simulink library "halout"  (R2021b)
settings: Solver=VariableStepAuto  StartTime=0.0  StopTime=10.0  RelTol=1e-3
undefined symbols (not defined in the file): C_TASK_5MS_S, FALSE, KHAL_CAN1FD1APS3E2E_flg, KHAL_CAN1FD1APS3TxReq_flg, KHAL_CAN1FD1VCU2E2E_flg, KHAL_CAN1FD1VCU2TxReq_flg, KHAL_CAN1FD1VCU3E2E_flg, KHAL_CAN1FD1VCU3TxReq_flg, KHAL_CAN1TxReq_flg, KHAL_CAN1VMCFCM1E2E_flg, KHAL_CAN1VMCFCM1TxReq_flg, KHAL_CAN2TxReq_flg, KHAL_CAN3FD3VCU1toNIDECTxReq_flg, KHAL_CAN3FD3VCU1TxReq_flg, KHAL_CAN3FD3VCU2E2E_flg, KHAL_CAN3FD3VCU2toNIDECE2E_flg, KHAL_CAN3FD3VCU2toNIDECTxReq_flg, KHAL_CAN3FD3VCU2TxReq_flg, KHAL_CAN3TxReq_flg, KHAL_CAN4FD4CE1000E2E_flg, KHAL_CAN4FD4CE1000TxReq_flg, KHAL_CAN4TxReq_flg, KHAL_CAN5TxReq_flg, KHAL_CAN6FD6APS3E2E_flg, KHAL_CAN6FD6APS3TxReq_flg, KHAL_CAN6FD6VCU2E2E_flg, KHAL_CAN6FD6VCU2TxReq_flg, KHAL_CAN6TxReq_flg, ONE_INT, TRUE, ZERO_INT
libraries: FVT_lib x500, simulink x235
(part 6 of 25)

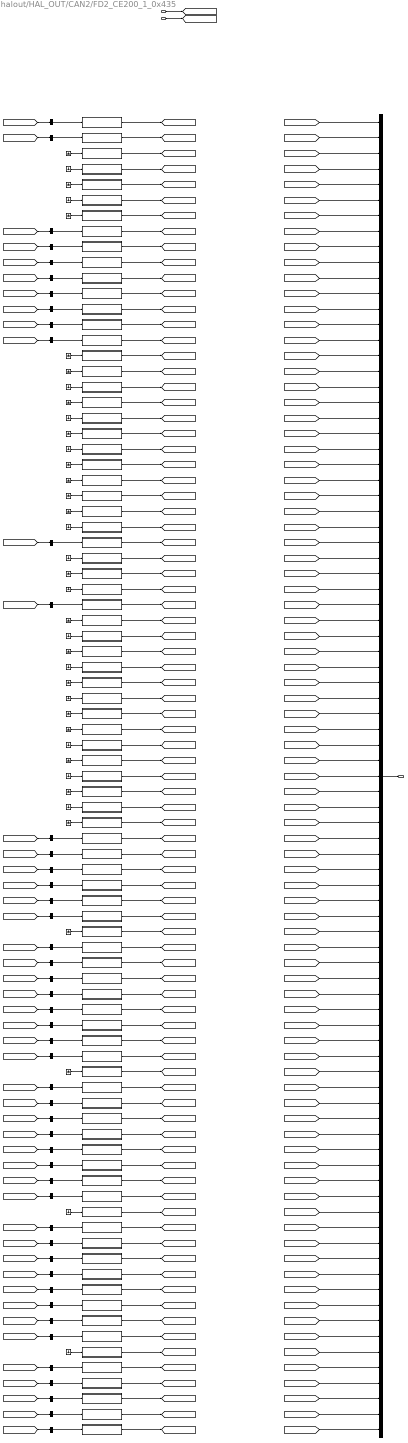
== system halout/HAL_OUT/CAN2/FD2_CE200_1_0x435 ==
  BSCP_outputs : Inport  OutDataTypeStr=Bus: BSCP_outputs
  BOUTP_outputs : Inport  Port=2  OutDataTypeStr=Bus: BOUTP_outputs
  AutoLTips : Subsystem
  CWheelTips : Subsystem
  FDCBCMAcc1StaSta : Subsystem
  FDCBCMAcc2StaSta : Subsystem
  FDCBCMAcc3StaSta : Subsystem
  FDCBCMAcc4StaSta : Subsystem
  FDCBCMAcc5StaSta : Subsystem
  FDCBCMAmbBrightStaSta : Subsystem
  FDCBCMAmbColorStaSta : Subsystem
  FDCBCMAmbDimENSta : Subsystem
  FDCBCMAmbFunENSta : Subsystem
  FDCBCMAmbLinkDriStaSta : Subsystem
  FDCBCMAmbODAENSta : Subsystem
  FDCBCMAmbPwrWarnENSta : Subsystem
  FDCBCMAmbWelENSta : Subsystem
  FDCBCMCLWinLockDrSta : Subsystem
  FDCBCMFollowMeENFunSta : Subsystem
  FDCBCMKey10AccSta : Subsystem
  FDCBCMKey1AccSta : Subsystem
  FDCBCMKey2AccSta : Subsystem
  FDCBCMKey3AccSta : Subsystem
  FDCBCMKey4AccSta : Subsystem
  FDCBCMKey5AccSta : Subsystem
  FDCBCMKey6AccSta : Subsystem
  FDCBCMKey7AccSta : Subsystem
  FDCBCMKey8AccSta : Subsystem
  FDCBCMKey9AccSta : Subsystem
  FDCBCMLockAlarmCmd : Subsystem
  FDCBCMPTGOpenHeightSta : Subsystem
  FDCBCMRmLpModeENFunSta : Subsystem
  FDCBCMTurnSwTSetStaSta : Subsystem
  FDCBCMUserNowSta : Subsystem
  FDCBCMWalkInUnLkEnFunSta : Subsystem
  FDCBCMWalkOutLkEnFunSta : Subsystem
  FDCDKCDkeyShowIVISta : Subsystem
  FDCDKCKeyMissSta : Subsystem
  FDCDKCKeyNumSta : Subsystem
  FDCDKCKeyTypeSta : Subsystem
  FDCDKCUIDLowPowerSta : Subsystem
  FDCFGSAirIntSta : Subsystem
  FDCFGSFGSChSta : Subsystem
  FDCFGSIONSWSta : Subsystem
  FDCSPTGSPTGENFunSta : Subsystem
  FDCTHCMAPTCForceOFFSta : Subsystem
  FDCTHCMAPTCWarningSta : Subsystem
  FDCTHCMAirIntZ3Sta : Subsystem
  Ground{,1..37} (38 alike) : Ground
  LFBatWarn : Subsystem
  LFPressIndi : Subsystem
  LFSensorFail : Subsystem
  LFWheelDebug : Subsystem
  LFWheelPSW : Subsystem
  LFWheelPress : Subsystem
  LFWheelShield : Subsystem
  LFWheelTemp : Subsystem
  LFWheelTmpIndi : Subsystem
  LRBatWarn : Subsystem
  LRPressIndi : Subsystem
  LRSensorFail : Subsystem
  LRWheelDebug : Subsystem
  LRWheelPSW : Subsystem
  LRWheelPress : Subsystem
  LRWheelShield : Subsystem
  LRWheelTemp : Subsystem
  LRWheelTmpIndi : Subsystem
  RFBatWarn : Subsystem
  RFPressIndi : Subsystem
  RFSensorFail : Subsystem
  RFWheelDebug : Subsystem
  RFWheelPSW : Subsystem
  RFWheelPress : Subsystem
  RFWheelShield : Subsystem
  RFWheelTemp : Subsystem
  RFWheelTmpIndi : Subsystem
  RRBatWarn : Subsystem
  RRPressIndi : Subsystem
  RRSensorFail : Subsystem
  RRWheelDebug : Subsystem
  RRWheelPSW : Subsystem
  RRWheelPress : Subsystem
  RRWheelShield : Subsystem
  RRWheelTemp : Subsystem
  RRWheelTmpIndi : Subsystem
  TPMSCaliButtAllow : Subsystem
  TPMSResButtAllow : Subsystem
  TPMSWarnIndi : Subsystem
  bus_creator : BusCreator  Inputs=85  OutDataTypeStr=Bus: DT_CAN2_SG_FD2_CE200_1  NonVirtualBus=on
  bus_selector : BusSelector  OutputSignals=VOUTP_AutoLTips_enum
  bus_selector1 : BusSelector  OutputSignals=VOUTP_CWheelTips_enum
  bus_selector10 : BusSelector  OutputSignals=VOUTP_LockAlarm_enum
  bus_selector11 : BusSelector  OutputSignals=VOUTP_UserNow_enum
  bus_selector12 : BusSelector  OutputSignals=VOUTP_LFBatWarn_flg
  bus_selector13 : BusSelector  OutputSignals=VOUTP_LFPressIndi_enum
  bus_selector14 : BusSelector  OutputSignals=VOUTP_LFSensorFail_flg
  bus_selector15 : BusSelector  OutputSignals=VOUTP_LFWheelDebug_flg
  bus_selector16 : BusSelector  OutputSignals=VOUTP_LFWheelPSW_raw8
  bus_selector17 : BusSelector  OutputSignals=VOUTP_LFWheelPress_raw8
  bus_selector18 : BusSelector  OutputSignals=VOUTP_LFWheelTemp_C
  bus_selector19 : BusSelector  OutputSignals=VOUTP_LFWheelTmpIndi_flg
  bus_selector2 : BusSelector  OutputSignals=VOUTP_AmbBrightSta_enum
  bus_selector20 : BusSelector  OutputSignals=VOUTP_LRBatWarn_flg
  bus_selector21 : BusSelector  OutputSignals=VOUTP_LRPressIndi_enum
  bus_selector22 : BusSelector  OutputSignals=VOUTP_LRSensorFail_flg
  bus_selector23 : BusSelector  OutputSignals=VOUTP_LRWheelDebug_flg
  bus_selector24 : BusSelector  OutputSignals=VOUTP_LRWheelPSW_raw8
  bus_selector25 : BusSelector  OutputSignals=VOUTP_LRWheelPress_raw8
  bus_selector26 : BusSelector  OutputSignals=VOUTP_LRWheelTemp_C
  bus_selector27 : BusSelector  OutputSignals=VOUTP_LRWheelTmpIndi_flg
  bus_selector28 : BusSelector  OutputSignals=VOUTP_RFBatWarn_flg
  bus_selector29 : BusSelector  OutputSignals=VOUTP_RFPressIndi_enum
  bus_selector3 : BusSelector  OutputSignals=VOUTP_AmbColorSta_enum
  bus_selector30 : BusSelector  OutputSignals=VOUTP_RFSensorFail_flg
  bus_selector31 : BusSelector  OutputSignals=VOUTP_RFWheelDebug_flg
  bus_selector32 : BusSelector  OutputSignals=VOUTP_RFWheelPSW_raw8
  bus_selector33 : BusSelector  OutputSignals=VOUTP_RFWheelPress_raw8
  bus_selector34 : BusSelector  OutputSignals=VOUTP_RFWheelTemp_C
  bus_selector35 : BusSelector  OutputSignals=VOUTP_RFWheelTmpIndi_flg
  bus_selector36 : BusSelector  OutputSignals=VOUTP_RRBatWarn_flg
  bus_selector37 : BusSelector  OutputSignals=VOUTP_RRPressIndi_enum
  bus_selector38 : BusSelector  OutputSignals=VOUTP_RRSensorFail_flg
  bus_selector39 : BusSelector  OutputSignals=VOUTP_RRWheelDebug_flg
  bus_selector4 : BusSelector  OutputSignals=VOUTP_AmbDimEN_flg
  bus_selector40 : BusSelector  OutputSignals=VOUTP_RRWheelPSW_raw8
  bus_selector41 : BusSelector  OutputSignals=VOUTP_RRWheelPress_raw8
  bus_selector42 : BusSelector  OutputSignals=VOUTP_RRWheelTemp_C
  bus_selector43 : BusSelector  OutputSignals=VOUTP_RRWheelTmpIndi_flg
  bus_selector44 : BusSelector  OutputSignals=VOUTP_TPMSWarnIndi_enum
  bus_selector45 : BusSelector  OutputSignals=VOUTP_TPMSCaliButtAllow_flg
  bus_selector46 : BusSelector  OutputSignals=VOUTP_TPMSResButtAllow_flg
  bus_selector5 : BusSelector  OutputSignals=VOUTP_AmbFunEN_flg
  bus_selector6 : BusSelector  OutputSignals=VOUTP_AmbLinkDriSta_flg
  bus_selector7 : BusSelector  OutputSignals=VOUTP_AmbODAEN_flg
  bus_selector8 : BusSelector  OutputSignals=VOUTP_AmbPwrWarnEN_flg
  bus_selector9 : BusSelector  OutputSignals=VOUTP_AmbWelEN_flg
  FD2_CE200_1 : Outport
  wires:
  BSCP_outputs/1 -> [BSCP_outputs]
  BOUTP_outputs/1 -> [BOUTP_outputs]
  [CAN2_AutoLTips] -> bus_creator/1  "CAN2_AutoLTips"
  [CAN2_CWheelTips] -> bus_creator/2  "CAN2_CWheelTips"
  [CAN2_FDC_BCM_Acc1Sta_Sta] -> bus_creator/3  "CAN2_FDC_BCM_Acc1Sta_Sta"
  [CAN2_FDC_BCM_Acc2Sta_Sta] -> bus_creator/4  "CAN2_FDC_BCM_Acc2Sta_Sta"
  [CAN2_FDC_BCM_Acc3Sta_Sta] -> bus_creator/5  "CAN2_FDC_BCM_Acc3Sta_Sta"
  [CAN2_FDC_BCM_Acc4Sta_Sta] -> bus_creator/6  "CAN2_FDC_BCM_Acc4Sta_Sta"
  [CAN2_FDC_BCM_Acc5Sta_Sta] -> bus_creator/7  "CAN2_FDC_BCM_Acc5Sta_Sta"
  [CAN2_FDC_BCM_AmbBrightSta_Sta] -> bus_creator/8  "CAN2_FDC_BCM_AmbBrightSta_Sta"
  [CAN2_FDC_BCM_AmbColorSta_Sta] -> bus_creator/9  "CAN2_FDC_BCM_AmbColorSta_Sta"
  [CAN2_FDC_BCM_AmbDimEN_Sta] -> bus_creator/10  "CAN2_FDC_BCM_AmbDimEN_Sta"
  [CAN2_FDC_BCM_AmbFunEN_Sta] -> bus_creator/11  "CAN2_FDC_BCM_AmbFunEN_Sta"
  [CAN2_FDC_BCM_AmbLinkDriSta_Sta] -> bus_creator/12  "CAN2_FDC_BCM_AmbLinkDriSta_Sta"
  [CAN2_FDC_BCM_AmbODAEN_Sta] -> bus_creator/13  "CAN2_FDC_BCM_AmbODAEN_Sta"
  [CAN2_FDC_BCM_AmbPwrWarnEN_Sta] -> bus_creator/14  "CAN2_FDC_BCM_AmbPwrWarnEN_Sta"
  [CAN2_FDC_BCM_AmbWelEN_Sta] -> bus_creator/15  "CAN2_FDC_BCM_AmbWelEN_Sta"
  [CAN2_FDC_BCM_CLWinLockDr_Sta] -> bus_creator/16  "CAN2_FDC_BCM_CLWinLockDr_Sta"
  [CAN2_FDC_BCM_FollowMeENFun_Sta] -> bus_creator/17  "CAN2_FDC_BCM_FollowMeENFun_Sta"
  [CAN2_FDC_BCM_Key10Acc_Sta] -> bus_creator/18  "CAN2_FDC_BCM_Key10Acc_Sta"
  [CAN2_FDC_BCM_Key1Acc_Sta] -> bus_creator/19  "CAN2_FDC_BCM_Key1Acc_Sta"
  [CAN2_FDC_BCM_Key2Acc_Sta] -> bus_creator/20  "CAN2_FDC_BCM_Key2Acc_Sta"
  [CAN2_FDC_BCM_Key3Acc_Sta] -> bus_creator/21  "CAN2_FDC_BCM_Key3Acc_Sta"
  [CAN2_FDC_BCM_Key4Acc_Sta] -> bus_creator/22  "CAN2_FDC_BCM_Key4Acc_Sta"
  [CAN2_FDC_BCM_Key5Acc_Sta] -> bus_creator/23  "CAN2_FDC_BCM_Key5Acc_Sta"
  [CAN2_FDC_BCM_Key6Acc_Sta] -> bus_creator/24  "CAN2_FDC_BCM_Key6Acc_Sta"
  [CAN2_FDC_BCM_Key7Acc_Sta] -> bus_creator/25  "CAN2_FDC_BCM_Key7Acc_Sta"
  [CAN2_FDC_BCM_Key8Acc_Sta] -> bus_creator/26  "CAN2_FDC_BCM_Key8Acc_Sta"
  [CAN2_FDC_BCM_Key9Acc_Sta] -> bus_creator/27  "CAN2_FDC_BCM_Key9Acc_Sta"
  [CAN2_FDC_BCM_LockAlarm_Cmd] -> bus_creator/28  "CAN2_FDC_BCM_LockAlarm_Cmd"
  [CAN2_FDC_BCM_PTGOpenHeight_Sta] -> bus_creator/29  "CAN2_FDC_BCM_PTGOpenHeight_Sta"
  [CAN2_FDC_BCM_RmLpModeENFun_Sta] -> bus_creator/30  "CAN2_FDC_BCM_RmLpModeENFun_Sta"
  [CAN2_FDC_BCM_TurnSwTSetSta_Sta] -> bus_creator/31  "CAN2_FDC_BCM_TurnSwTSetSta_Sta"
  [CAN2_FDC_BCM_UserNow_Sta] -> bus_creator/32  "CAN2_FDC_BCM_UserNow_Sta"
  [CAN2_FDC_BCM_WalkInUnLkEnFun_Sta] -> bus_creator/33  "CAN2_FDC_BCM_WalkInUnLkEnFun_Sta"
  [CAN2_FDC_BCM_WalkOutLkEnFun_Sta] -> bus_creator/34  "CAN2_FDC_BCM_WalkOutLkEnFun_Sta"
  [CAN2_FDC_DKC_DkeyShowIVI_Sta] -> bus_creator/35  "CAN2_FDC_DKC_DkeyShowIVI_Sta"
  [CAN2_FDC_DKC_KeyMiss_Sta] -> bus_creator/36  "CAN2_FDC_DKC_KeyMiss_Sta"
  [CAN2_FDC_DKC_KeyNum_Sta] -> bus_creator/37  "CAN2_FDC_DKC_KeyNum_Sta"
  [CAN2_FDC_DKC_KeyType_Sta] -> bus_creator/38  "CAN2_FDC_DKC_KeyType_Sta"
  [CAN2_FDC_DKC_UIDLowPower_Sta] -> bus_creator/39  "CAN2_FDC_DKC_UIDLowPower_Sta"
  [CAN2_FDC_FGS_AirInt_Sta] -> bus_creator/40  "CAN2_FDC_FGS_AirInt_Sta"
  [CAN2_FDC_FGS_FGSCh_Sta] -> bus_creator/41  "CAN2_FDC_FGS_FGSCh_Sta"
  [CAN2_FDC_FGS_IONSW_Sta] -> bus_creator/42  "CAN2_FDC_FGS_IONSW_Sta"
  [CAN2_FDC_SPTG_SPTGENFun_Sta] -> bus_creator/43  "CAN2_FDC_SPTG_SPTGENFun_Sta"
  [CAN2_FDC_THCM_APTCForceOFF_Sta] -> bus_creator/44  "CAN2_FDC_THCM_APTCForceOFF_Sta"
  [CAN2_FDC_THCM_APTCWarning_Sta] -> bus_creator/45  "CAN2_FDC_THCM_APTCWarning_Sta"
  [CAN2_FDC_THCM_AirIntZ3_Sta] -> bus_creator/46  "CAN2_FDC_THCM_AirIntZ3_Sta"
  [CAN2_LFBatWarn] -> bus_creator/47  "CAN2_LFBatWarn"
  [CAN2_LFPressIndi] -> bus_creator/48  "CAN2_LFPressIndi"
  [CAN2_LFSensorFail] -> bus_creator/49  "CAN2_LFSensorFail"
  [CAN2_LFWheelDebug] -> bus_creator/50  "CAN2_LFWheelDebug"
  [CAN2_LFWheelPSW] -> bus_creator/51  "CAN2_LFWheelPSW"
  [CAN2_LFWheelPress] -> bus_creator/52  "CAN2_LFWheelPress"
  [CAN2_LFWheelShield] -> bus_creator/53  "CAN2_LFWheelShield"
  [CAN2_LFWheelTemp] -> bus_creator/54  "CAN2_LFWheelTemp"
  [CAN2_LFWheelTmpIndi] -> bus_creator/55  "CAN2_LFWheelTmpIndi"
  [CAN2_LRBatWarn] -> bus_creator/56  "CAN2_LRBatWarn"
  [CAN2_LRPressIndi] -> bus_creator/57  "CAN2_LRPressIndi"
  [CAN2_LRSensorFail] -> bus_creator/58  "CAN2_LRSensorFail"
  [CAN2_LRWheelDebug] -> bus_creator/59  "CAN2_LRWheelDebug"
  [CAN2_LRWheelPSW] -> bus_creator/60  "CAN2_LRWheelPSW"
  [CAN2_LRWheelPress] -> bus_creator/61  "CAN2_LRWheelPress"
  [CAN2_LRWheelShield] -> bus_creator/62  "CAN2_LRWheelShield"
  [CAN2_LRWheelTemp] -> bus_creator/63  "CAN2_LRWheelTemp"
  [CAN2_LRWheelTmpIndi] -> bus_creator/64  "CAN2_LRWheelTmpIndi"
  [CAN2_RFBatWarn] -> bus_creator/65  "CAN2_RFBatWarn"
  [CAN2_RFPressIndi] -> bus_creator/66  "CAN2_RFPressIndi"
  [CAN2_RFSensorFail] -> bus_creator/67  "CAN2_RFSensorFail"
  [CAN2_RFWheelDebug] -> bus_creator/68  "CAN2_RFWheelDebug"
  [CAN2_RFWheelPSW] -> bus_creator/69  "CAN2_RFWheelPSW"
  [CAN2_RFWheelPress] -> bus_creator/70  "CAN2_RFWheelPress"
  [CAN2_RFWheelShield] -> bus_creator/71  "CAN2_RFWheelShield"
  [CAN2_RFWheelTemp] -> bus_creator/72  "CAN2_RFWheelTemp"
  [CAN2_RFWheelTmpIndi] -> bus_creator/73  "CAN2_RFWheelTmpIndi"
  [CAN2_RRBatWarn] -> bus_creator/74  "CAN2_RRBatWarn"
  [CAN2_RRPressIndi] -> bus_creator/75  "CAN2_RRPressIndi"
  [CAN2_RRSensorFail] -> bus_creator/76  "CAN2_RRSensorFail"
  [CAN2_RRWheelDebug] -> bus_creator/77  "CAN2_RRWheelDebug"
  [CAN2_RRWheelPSW] -> bus_creator/78  "CAN2_RRWheelPSW"
  [CAN2_RRWheelPress] -> bus_creator/79  "CAN2_RRWheelPress"
  [CAN2_RRWheelShield] -> bus_creator/80  "CAN2_RRWheelShield"
  [CAN2_RRWheelTemp] -> bus_creator/81  "CAN2_RRWheelTemp"
  [CAN2_RRWheelTmpIndi] -> bus_creator/82  "CAN2_RRWheelTmpIndi"
  [CAN2_TPMSWarnIndi] -> bus_creator/83  "CAN2_TPMSWarnIndi"
  [CAN2_TPMS_Cali_Butt_Allow] -> bus_creator/84  "CAN2_TPMS_Cali_Butt_Allow"
  [CAN2_TPMS_Res_Butt_Allow] -> bus_creator/85  "CAN2_TPMS_Res_Butt_Allow"
  bus_creator/1 -> FD2_CE200_1/1
  AutoLTips/1(CAN2_AutoLTips) -> [CAN2_AutoLTips]
  CWheelTips/1(CAN2_CWheelTips) -> [CAN2_CWheelTips]
  FDCBCMAcc1StaSta/1(CAN2_FDC_BCM_Acc1Sta_Sta) -> [CAN2_FDC_BCM_Acc1Sta_Sta]
  FDCBCMAcc2StaSta/1(CAN2_FDC_BCM_Acc2Sta_Sta) -> [CAN2_FDC_BCM_Acc2Sta_Sta]
  FDCBCMAcc3StaSta/1(CAN2_FDC_BCM_Acc3Sta_Sta) -> [CAN2_FDC_BCM_Acc3Sta_Sta]
  FDCBCMAcc4StaSta/1(CAN2_FDC_BCM_Acc4Sta_Sta) -> [CAN2_FDC_BCM_Acc4Sta_Sta]
  FDCBCMAcc5StaSta/1(CAN2_FDC_BCM_Acc5Sta_Sta) -> [CAN2_FDC_BCM_Acc5Sta_Sta]
  FDCBCMAmbBrightStaSta/1(CAN2_FDC_BCM_AmbBrightSta_Sta) -> [CAN2_FDC_BCM_AmbBrightSta_Sta]
  FDCBCMAmbColorStaSta/1(CAN2_FDC_BCM_AmbColorSta_Sta) -> [CAN2_FDC_BCM_AmbColorSta_Sta]
  FDCBCMAmbDimENSta/1(CAN2_FDC_BCM_AmbDimEN_Sta) -> [CAN2_FDC_BCM_AmbDimEN_Sta]
  FDCBCMAmbFunENSta/1(CAN2_FDC_BCM_AmbFunEN_Sta) -> [CAN2_FDC_BCM_AmbFunEN_Sta]
  FDCBCMAmbLinkDriStaSta/1(CAN2_FDC_BCM_AmbLinkDriSta_Sta) -> [CAN2_FDC_BCM_AmbLinkDriSta_Sta]
  FDCBCMAmbODAENSta/1(CAN2_FDC_BCM_AmbODAEN_Sta) -> [CAN2_FDC_BCM_AmbODAEN_Sta]
  FDCBCMAmbPwrWarnENSta/1(CAN2_FDC_BCM_AmbPwrWarnEN_Sta) -> [CAN2_FDC_BCM_AmbPwrWarnEN_Sta]
  FDCBCMAmbWelENSta/1(CAN2_FDC_BCM_AmbWelEN_Sta) -> [CAN2_FDC_BCM_AmbWelEN_Sta]
  FDCBCMCLWinLockDrSta/1(CAN2_FDC_BCM_CLWinLockDr_Sta) -> [CAN2_FDC_BCM_CLWinLockDr_Sta]
  FDCBCMFollowMeENFunSta/1(CAN2_FDC_BCM_FollowMeENFun_Sta) -> [CAN2_FDC_BCM_FollowMeENFun_Sta]
  FDCBCMKey10AccSta/1(CAN2_FDC_BCM_Key10Acc_Sta) -> [CAN2_FDC_BCM_Key10Acc_Sta]
  FDCBCMKey1AccSta/1(CAN2_FDC_BCM_Key1Acc_Sta) -> [CAN2_FDC_BCM_Key1Acc_Sta]
  FDCBCMKey2AccSta/1(CAN2_FDC_BCM_Key2Acc_Sta) -> [CAN2_FDC_BCM_Key2Acc_Sta]
  FDCBCMKey3AccSta/1(CAN2_FDC_BCM_Key3Acc_Sta) -> [CAN2_FDC_BCM_Key3Acc_Sta]
  FDCBCMKey4AccSta/1(CAN2_FDC_BCM_Key4Acc_Sta) -> [CAN2_FDC_BCM_Key4Acc_Sta]
  FDCBCMKey5AccSta/1(CAN2_FDC_BCM_Key5Acc_Sta) -> [CAN2_FDC_BCM_Key5Acc_Sta]
  FDCBCMKey6AccSta/1(CAN2_FDC_BCM_Key6Acc_Sta) -> [CAN2_FDC_BCM_Key6Acc_Sta]
  FDCBCMKey7AccSta/1(CAN2_FDC_BCM_Key7Acc_Sta) -> [CAN2_FDC_BCM_Key7Acc_Sta]
  FDCBCMKey8AccSta/1(CAN2_FDC_BCM_Key8Acc_Sta) -> [CAN2_FDC_BCM_Key8Acc_Sta]
  FDCBCMKey9AccSta/1(CAN2_FDC_BCM_Key9Acc_Sta) -> [CAN2_FDC_BCM_Key9Acc_Sta]
  FDCBCMLockAlarmCmd/1(CAN2_FDC_BCM_LockAlarm_Cmd) -> [CAN2_FDC_BCM_LockAlarm_Cmd]
  FDCBCMPTGOpenHeightSta/1(CAN2_FDC_BCM_PTGOpenHeight_Sta) -> [CAN2_FDC_BCM_PTGOpenHeight_Sta]
  FDCBCMRmLpModeENFunSta/1(CAN2_FDC_BCM_RmLpModeENFun_Sta) -> [CAN2_FDC_BCM_RmLpModeENFun_Sta]
  FDCBCMTurnSwTSetStaSta/1(CAN2_FDC_BCM_TurnSwTSetSta_Sta) -> [CAN2_FDC_BCM_TurnSwTSetSta_Sta]
  FDCBCMUserNowSta/1(CAN2_FDC_BCM_UserNow_Sta) -> [CAN2_FDC_BCM_UserNow_Sta]
  FDCBCMWalkInUnLkEnFunSta/1(CAN2_FDC_BCM_WalkInUnLkEnFun_Sta) -> [CAN2_FDC_BCM_WalkInUnLkEnFun_Sta]
  FDCBCMWalkOutLkEnFunSta/1(CAN2_FDC_BCM_WalkOutLkEnFun_Sta) -> [CAN2_FDC_BCM_WalkOutLkEnFun_Sta]
  FDCDKCDkeyShowIVISta/1(CAN2_FDC_DKC_DkeyShowIVI_Sta) -> [CAN2_FDC_DKC_DkeyShowIVI_Sta]
  FDCDKCKeyMissSta/1(CAN2_FDC_DKC_KeyMiss_Sta) -> [CAN2_FDC_DKC_KeyMiss_Sta]
  FDCDKCKeyNumSta/1(CAN2_FDC_DKC_KeyNum_Sta) -> [CAN2_FDC_DKC_KeyNum_Sta]
  FDCDKCKeyTypeSta/1(CAN2_FDC_DKC_KeyType_Sta) -> [CAN2_FDC_DKC_KeyType_Sta]
  FDCDKCUIDLowPowerSta/1(CAN2_FDC_DKC_UIDLowPower_Sta) -> [CAN2_FDC_DKC_UIDLowPower_Sta]
  FDCFGSAirIntSta/1(CAN2_FDC_FGS_AirInt_Sta) -> [CAN2_FDC_FGS_AirInt_Sta]
  FDCFGSFGSChSta/1(CAN2_FDC_FGS_FGSCh_Sta) -> [CAN2_FDC_FGS_FGSCh_Sta]
  FDCFGSIONSWSta/1(CAN2_FDC_FGS_IONSW_Sta) -> [CAN2_FDC_FGS_IONSW_Sta]
  FDCSPTGSPTGENFunSta/1(CAN2_FDC_SPTG_SPTGENFun_Sta) -> [CAN2_FDC_SPTG_SPTGENFun_Sta]
  FDCTHCMAPTCForceOFFSta/1(CAN2_FDC_THCM_APTCForceOFF_Sta) -> [CAN2_FDC_THCM_APTCForceOFF_Sta]
  FDCTHCMAPTCWarningSta/1(CAN2_FDC_THCM_APTCWarning_Sta) -> [CAN2_FDC_THCM_APTCWarning_Sta]
  FDCTHCMAirIntZ3Sta/1(CAN2_FDC_THCM_AirIntZ3_Sta) -> [CAN2_FDC_THCM_AirIntZ3_Sta]
  LFBatWarn/1(CAN2_LFBatWarn) -> [CAN2_LFBatWarn]
  LFPressIndi/1(CAN2_LFPressIndi) -> [CAN2_LFPressIndi]
  LFSensorFail/1(CAN2_LFSensorFail) -> [CAN2_LFSensorFail]
  LFWheelDebug/1(CAN2_LFWheelDebug) -> [CAN2_LFWheelDebug]
  LFWheelPSW/1(CAN2_LFWheelPSW) -> [CAN2_LFWheelPSW]
  LFWheelPress/1(CAN2_LFWheelPress) -> [CAN2_LFWheelPress]
  LFWheelShield/1(CAN2_LFWheelShield) -> [CAN2_LFWheelShield]
  LFWheelTemp/1(CAN2_LFWheelTemp) -> [CAN2_LFWheelTemp]
  LFWheelTmpIndi/1(CAN2_LFWheelTmpIndi) -> [CAN2_LFWheelTmpIndi]
  LRBatWarn/1(CAN2_LRBatWarn) -> [CAN2_LRBatWarn]
  LRPressIndi/1(CAN2_LRPressIndi) -> [CAN2_LRPressIndi]
  LRSensorFail/1(CAN2_LRSensorFail) -> [CAN2_LRSensorFail]
  LRWheelDebug/1(CAN2_LRWheelDebug) -> [CAN2_LRWheelDebug]
  LRWheelPSW/1(CAN2_LRWheelPSW) -> [CAN2_LRWheelPSW]
  LRWheelPress/1(CAN2_LRWheelPress) -> [CAN2_LRWheelPress]
  LRWheelShield/1(CAN2_LRWheelShield) -> [CAN2_LRWheelShield]
  LRWheelTemp/1(CAN2_LRWheelTemp) -> [CAN2_LRWheelTemp]
  LRWheelTmpIndi/1(CAN2_LRWheelTmpIndi) -> [CAN2_LRWheelTmpIndi]
  RFBatWarn/1(CAN2_RFBatWarn) -> [CAN2_RFBatWarn]
  RFPressIndi/1(CAN2_RFPressIndi) -> [CAN2_RFPressIndi]
  RFSensorFail/1(CAN2_RFSensorFail) -> [CAN2_RFSensorFail]
  RFWheelDebug/1(CAN2_RFWheelDebug) -> [CAN2_RFWheelDebug]
  RFWheelPSW/1(CAN2_RFWheelPSW) -> [CAN2_RFWheelPSW]
  RFWheelPress/1(CAN2_RFWheelPress) -> [CAN2_RFWheelPress]
  RFWheelShield/1(CAN2_RFWheelShield) -> [CAN2_RFWheelShield]
  RFWheelTemp/1(CAN2_RFWheelTemp) -> [CAN2_RFWheelTemp]
  RFWheelTmpIndi/1(CAN2_RFWheelTmpIndi) -> [CAN2_RFWheelTmpIndi]
  RRBatWarn/1(CAN2_RRBatWarn) -> [CAN2_RRBatWarn]
  RRPressIndi/1(CAN2_RRPressIndi) -> [CAN2_RRPressIndi]
  RRSensorFail/1(CAN2_RRSensorFail) -> [CAN2_RRSensorFail]
  RRWheelDebug/1(CAN2_RRWheelDebug) -> [CAN2_RRWheelDebug]
  RRWheelPSW/1(CAN2_RRWheelPSW) -> [CAN2_RRWheelPSW]
  RRWheelPress/1(CAN2_RRWheelPress) -> [CAN2_RRWheelPress]
  RRWheelShield/1(CAN2_RRWheelShield) -> [CAN2_RRWheelShield]
  RRWheelTemp/1(CAN2_RRWheelTemp) -> [CAN2_RRWheelTemp]
  RRWheelTmpIndi/1(CAN2_RRWheelTmpIndi) -> [CAN2_RRWheelTmpIndi]
  TPMSWarnIndi/1(CAN2_TPMSWarnIndi) -> [CAN2_TPMSWarnIndi]
  TPMSCaliButtAllow/1(CAN2_TPMS_Cali_Butt_Allow) -> [CAN2_TPMS_Cali_Butt_Allow]
  TPMSResButtAllow/1(CAN2_TPMS_Res_Butt_Allow) -> [CAN2_TPMS_Res_Butt_Allow]
  bus_selector/1 -> AutoLTips/1(AutoLTips)  "<VOUTP_AutoLTips_enum>"
  [BOUTP_outputs] -> bus_selector/1
  bus_selector1/1 -> CWheelTips/1(CWheelTips)  "<VOUTP_CWheelTips_enum>"
  [BOUTP_outputs] -> bus_selector1/1
  Ground/1 -> FDCBCMAcc1StaSta/1(FDCBCMAcc1StaSta)
  Ground1/1 -> FDCBCMAcc2StaSta/1(FDCBCMAcc2StaSta)
  Ground2/1 -> FDCBCMAcc3StaSta/1(FDCBCMAcc3StaSta)
  Ground3/1 -> FDCBCMAcc4StaSta/1(FDCBCMAcc4StaSta)
  Ground4/1 -> FDCBCMAcc5StaSta/1(FDCBCMAcc5StaSta)
  bus_selector2/1 -> FDCBCMAmbBrightStaSta/1(FDCBCMAmbBrightStaSta)  "<VOUTP_AmbBrightSta_enum>"
  [BOUTP_outputs] -> bus_selector2/1
  bus_selector3/1 -> FDCBCMAmbColorStaSta/1(FDCBCMAmbColorStaSta)  "<VOUTP_AmbColorSta_enum>"
  [BOUTP_outputs] -> bus_selector3/1
  bus_selector4/1 -> FDCBCMAmbDimENSta/1(FDCBCMAmbDimENSta)  "<VOUTP_AmbDimEN_flg>"
  [BOUTP_outputs] -> bus_selector4/1
  bus_selector5/1 -> FDCBCMAmbFunENSta/1(FDCBCMAmbFunENSta)  "<VOUTP_AmbFunEN_flg>"
  [BOUTP_outputs] -> bus_selector5/1
  bus_selector6/1 -> FDCBCMAmbLinkDriStaSta/1(FDCBCMAmbLinkDriStaSta)  "<VOUTP_AmbLinkDriSta_flg>"
  [BOUTP_outputs] -> bus_selector6/1
  bus_selector7/1 -> FDCBCMAmbODAENSta/1(FDCBCMAmbODAENSta)  "<VOUTP_AmbODAEN_flg>"
  [BOUTP_outputs] -> bus_selector7/1
  bus_selector8/1 -> FDCBCMAmbPwrWarnENSta/1(FDCBCMAmbPwrWarnENSta)  "<VOUTP_AmbPwrWarnEN_flg>"
  [BOUTP_outputs] -> bus_selector8/1
  bus_selector9/1 -> FDCBCMAmbWelENSta/1(FDCBCMAmbWelENSta)  "<VOUTP_AmbWelEN_flg>"
  [BOUTP_outputs] -> bus_selector9/1
  Ground5/1 -> FDCBCMCLWinLockDrSta/1(FDCBCMCLWinLockDrSta)
  Ground6/1 -> FDCBCMFollowMeENFunSta/1(FDCBCMFollowMeENFunSta)
  Ground7/1 -> FDCBCMKey10AccSta/1(FDCBCMKey10AccSta)
  Ground8/1 -> FDCBCMKey1AccSta/1(FDCBCMKey1AccSta)
  Ground9/1 -> FDCBCMKey2AccSta/1(FDCBCMKey2AccSta)
  Ground10/1 -> FDCBCMKey3AccSta/1(FDCBCMKey3AccSta)
  Ground11/1 -> FDCBCMKey4AccSta/1(FDCBCMKey4AccSta)
  Ground12/1 -> FDCBCMKey5AccSta/1(FDCBCMKey5AccSta)
  Ground13/1 -> FDCBCMKey6AccSta/1(FDCBCMKey6AccSta)
  Ground14/1 -> FDCBCMKey7AccSta/1(FDCBCMKey7AccSta)
  Ground15/1 -> FDCBCMKey8AccSta/1(FDCBCMKey8AccSta)
  Ground16/1 -> FDCBCMKey9AccSta/1(FDCBCMKey9AccSta)
  bus_selector10/1 -> FDCBCMLockAlarmCmd/1(FDCBCMLockAlarmCmd)  "<VOUTP_LockAlarm_enum>"
  [BOUTP_outputs] -> bus_selector10/1
  Ground17/1 -> FDCBCMPTGOpenHeightSta/1(FDCBCMPTGOpenHeightSta)
  Ground18/1 -> FDCBCMRmLpModeENFunSta/1(FDCBCMRmLpModeENFunSta)
  Ground19/1 -> FDCBCMTurnSwTSetStaSta/1(FDCBCMTurnSwTSetStaSta)
  bus_selector11/1 -> FDCBCMUserNowSta/1(FDCBCMUserNowSta)  "<VOUTP_UserNow_enum>"
  [BOUTP_outputs] -> bus_selector11/1
  Ground20/1 -> FDCBCMWalkInUnLkEnFunSta/1(FDCBCMWalkInUnLkEnFunSta)
  Ground21/1 -> FDCBCMWalkOutLkEnFunSta/1(FDCBCMWalkOutLkEnFunSta)
  Ground22/1 -> FDCDKCDkeyShowIVISta/1(FDCDKCDkeyShowIVISta)
  Ground23/1 -> FDCDKCKeyMissSta/1(FDCDKCKeyMissSta)
  Ground24/1 -> FDCDKCKeyNumSta/1(FDCDKCKeyNumSta)
  Ground25/1 -> FDCDKCKeyTypeSta/1(FDCDKCKeyTypeSta)
  Ground26/1 -> FDCDKCUIDLowPowerSta/1(FDCDKCUIDLowPowerSta)
  Ground27/1 -> FDCFGSAirIntSta/1(FDCFGSAirIntSta)
  Ground28/1 -> FDCFGSFGSChSta/1(FDCFGSFGSChSta)
  Ground29/1 -> FDCFGSIONSWSta/1(FDCFGSIONSWSta)
  Ground30/1 -> FDCSPTGSPTGENFunSta/1(FDCSPTGSPTGENFunSta)
  Ground31/1 -> FDCTHCMAPTCForceOFFSta/1(FDCTHCMAPTCForceOFFSta)
  Ground32/1 -> FDCTHCMAPTCWarningSta/1(FDCTHCMAPTCWarningSta)
  Ground33/1 -> FDCTHCMAirIntZ3Sta/1(FDCTHCMAirIntZ3Sta)
  bus_selector12/1 -> LFBatWarn/1(LFBatWarn)  "<VOUTP_LFBatWarn_flg>"
  [BOUTP_outputs] -> bus_selector12/1
  bus_selector13/1 -> LFPressIndi/1(LFPressIndi)  "<VOUTP_LFPressIndi_enum>"
  [BOUTP_outputs] -> bus_selector13/1
  bus_selector14/1 -> LFSensorFail/1(LFSensorFail)  "<VOUTP_LFSensorFail_flg>"
  [BOUTP_outputs] -> bus_selector14/1
  bus_selector15/1 -> LFWheelDebug/1(LFWheelDebug)  "<VOUTP_LFWheelDebug_flg>"
  [BOUTP_outputs] -> bus_selector15/1
  bus_selector16/1 -> LFWheelPSW/1(LFWheelPSW)  "<VOUTP_LFWheelPSW_raw8>"
  [BOUTP_outputs] -> bus_selector16/1
  bus_selector17/1 -> LFWheelPress/1(LFWheelPress)  "<VOUTP_LFWheelPress_raw8>"
  [BOUTP_outputs] -> bus_selector17/1
  Ground34/1 -> LFWheelShield/1(LFWheelShield)
  bus_selector18/1 -> LFWheelTemp/1(LFWheelTemp)  "<VOUTP_LFWheelTemp_C>"
  [BOUTP_outputs] -> bus_selector18/1
  bus_selector19/1 -> LFWheelTmpIndi/1(LFWheelTmpIndi)  "<VOUTP_LFWheelTmpIndi_flg>"
  [BOUTP_outputs] -> bus_selector19/1
  bus_selector20/1 -> LRBatWarn/1(LRBatWarn)  "<VOUTP_LRBatWarn_flg>"
  [BOUTP_outputs] -> bus_selector20/1
  bus_selector21/1 -> LRPressIndi/1(LRPressIndi)  "<VOUTP_LRPressIndi_enum>"
  [BOUTP_outputs] -> bus_selector21/1
  bus_selector22/1 -> LRSensorFail/1(LRSensorFail)  "<VOUTP_LRSensorFail_flg>"
  [BOUTP_outputs] -> bus_selector22/1
  bus_selector23/1 -> LRWheelDebug/1(LRWheelDebug)  "<VOUTP_LRWheelDebug_flg>"
  [BOUTP_outputs] -> bus_selector23/1
  bus_selector24/1 -> LRWheelPSW/1(LRWheelPSW)  "<VOUTP_LRWheelPSW_raw8>"
  [BOUTP_outputs] -> bus_selector24/1
  bus_selector25/1 -> LRWheelPress/1(LRWheelPress)  "<VOUTP_LRWheelPress_raw8>"
  [BOUTP_outputs] -> bus_selector25/1
  Ground35/1 -> LRWheelShield/1(LRWheelShield)
  bus_selector26/1 -> LRWheelTemp/1(LRWheelTemp)  "<VOUTP_LRWheelTemp_C>"
  [BOUTP_outputs] -> bus_selector26/1
  bus_selector27/1 -> LRWheelTmpIndi/1(LRWheelTmpIndi)  "<VOUTP_LRWheelTmpIndi_flg>"
  [BOUTP_outputs] -> bus_selector27/1
  bus_selector28/1 -> RFBatWarn/1(RFBatWarn)  "<VOUTP_RFBatWarn_flg>"
  [BOUTP_outputs] -> bus_selector28/1
  bus_selector29/1 -> RFPressIndi/1(RFPressIndi)  "<VOUTP_RFPressIndi_enum>"
  [BOUTP_outputs] -> bus_selector29/1
  bus_selector30/1 -> RFSensorFail/1(RFSensorFail)  "<VOUTP_RFSensorFail_flg>"
  [BOUTP_outputs] -> bus_selector30/1
  bus_selector31/1 -> RFWheelDebug/1(RFWheelDebug)  "<VOUTP_RFWheelDebug_flg>"
  [BOUTP_outputs] -> bus_selector31/1
  bus_selector32/1 -> RFWheelPSW/1(RFWheelPSW)  "<VOUTP_RFWheelPSW_raw8>"
  [BOUTP_outputs] -> bus_selector32/1
  bus_selector33/1 -> RFWheelPress/1(RFWheelPress)  "<VOUTP_RFWheelPress_raw8>"
  [BOUTP_outputs] -> bus_selector33/1
  Ground36/1 -> RFWheelShield/1(RFWheelShield)
  bus_selector34/1 -> RFWheelTemp/1(RFWheelTemp)  "<VOUTP_RFWheelTemp_C>"
  [BOUTP_outputs] -> bus_selector34/1
  bus_selector35/1 -> RFWheelTmpIndi/1(RFWheelTmpIndi)  "<VOUTP_RFWheelTmpIndi_flg>"
  [BOUTP_outputs] -> bus_selector35/1
  bus_selector36/1 -> RRBatWarn/1(RRBatWarn)  "<VOUTP_RRBatWarn_flg>"
  [BOUTP_outputs] -> bus_selector36/1
  bus_selector37/1 -> RRPressIndi/1(RRPressIndi)  "<VOUTP_RRPressIndi_enum>"
  [BOUTP_outputs] -> bus_selector37/1
  bus_selector38/1 -> RRSensorFail/1(RRSensorFail)  "<VOUTP_RRSensorFail_flg>"
  [BOUTP_outputs] -> bus_selector38/1
  bus_selector39/1 -> RRWheelDebug/1(RRWheelDebug)  "<VOUTP_RRWheelDebug_flg>"
  [BOUTP_outputs] -> bus_selector39/1
  bus_selector40/1 -> RRWheelPSW/1(RRWheelPSW)  "<VOUTP_RRWheelPSW_raw8>"
  [BOUTP_outputs] -> bus_selector40/1
  bus_selector41/1 -> RRWheelPress/1(RRWheelPress)  "<VOUTP_RRWheelPress_raw8>"
  [BOUTP_outputs] -> bus_selector41/1
  Ground37/1 -> RRWheelShield/1(RRWheelShield)
  bus_selector42/1 -> RRWheelTemp/1(RRWheelTemp)  "<VOUTP_RRWheelTemp_C>"
  [BOUTP_outputs] -> bus_selector42/1
  bus_selector43/1 -> RRWheelTmpIndi/1(RRWheelTmpIndi)  "<VOUTP_RRWheelTmpIndi_flg>"
  [BOUTP_outputs] -> bus_selector43/1
  bus_selector44/1 -> TPMSWarnIndi/1(TPMSWarnIndi)  "<VOUTP_TPMSWarnIndi_enum>"
  [BOUTP_outputs] -> bus_selector44/1
  bus_selector45/1 -> TPMSCaliButtAllow/1(TPMSCaliButtAllow)  "<VOUTP_TPMSCaliButtAllow_flg>"
  [BOUTP_outputs] -> bus_selector45/1
  bus_selector46/1 -> TPMSResButtAllow/1(TPMSResButtAllow)  "<VOUTP_TPMSResButtAllow_flg>"
  [BOUTP_outputs] -> bus_selector46/1

== system halout/HAL_OUT/CAN2/FD2_Version_0x3C3 ==
  BSCP_outputs : Inport  OutDataTypeStr=Bus: BSCP_outputs
  BOUTP_outputs : Inport  Port=2  OutDataTypeStr=Bus: BOUTP_outputs
  FUSIONHWVer1 : Subsystem
  FUSIONHWVer2 : Subsystem
  FUSIONHWVer3 : Subsystem
  FUSIONSWCarModel1 : Subsystem
  FUSIONSWCarModel2 : Subsystem
  FUSIONSWCarModel3 : Subsystem
  FUSIONSWController1 : Subsystem
  FUSIONSWController2 : Subsystem
  FUSIONSWCountry1 : Subsystem
  FUSIONSWCountry2 : Subsystem
  FUSIONSWECUGen1 : Subsystem
  FUSIONSWECUGen2 : Subsystem
  FUSIONSWMajor1 : Subsystem
  FUSIONSWMajor2 : Subsystem
  FUSIONSWMinor1 : Subsystem
  FUSIONSWMinor2 : Subsystem
  FUSIONSWPatch1 : Subsystem
  FUSIONSWPatch2 : Subsystem
  FUSIONSWSHA1 : Subsystem
  FUSIONSWSHA2 : Subsystem
  FUSIONSWSHA3 : Subsystem
  FUSIONSWSHA4 : Subsystem
  FUSIONSWSHA5 : Subsystem
  FUSIONSWSHA6 : Subsystem
  FUSIONSWSHA7 : Subsystem
  FUSIONSWSHA8 : Subsystem
  FUSIONSWVar1 : Subsystem
  FUSIONSWVar2 : Subsystem
  FUSIONSWVar3 : Subsystem
  FUSIONSWVar4 : Subsystem
  FUSIONSWVar5 : Subsystem
  FUSIONSWchange1 : Subsystem
  FUSIONSWchange2 : Subsystem
  FUSIONSWdash1 : Subsystem
  FUSIONSWdash2 : Subsystem
  Ground{,1..5} (6 alike) : Ground
  bus_creator : BusCreator  Inputs=35  OutDataTypeStr=Bus: DT_CAN2_SG_FD2_Version  NonVirtualBus=on
  bus_selector : BusSelector  OutputSignals=VOUTP_HWVer1_cnt
  bus_selector1 : BusSelector  OutputSignals=VOUTP_HWVer2_cnt
  bus_selector10 : BusSelector  OutputSignals=VOUTP_Major1_cnt
  bus_selector11 : BusSelector  OutputSignals=VOUTP_Major2_cnt
  bus_selector12 : BusSelector  OutputSignals=VOUTP_Minor1_cnt
  bus_selector13 : BusSelector  OutputSignals=VOUTP_Minor2_cnt
  bus_selector14 : BusSelector  OutputSignals=VOUTP_Patch1_cnt
  bus_selector15 : BusSelector  OutputSignals=VOUTP_Patch2_cnt
  bus_selector16 : BusSelector  OutputSignals=VOUTP_SHA1_cnt
  bus_selector17 : BusSelector  OutputSignals=VOUTP_SHA2_cnt
  bus_selector18 : BusSelector  OutputSignals=VOUTP_SHA3_cnt
  bus_selector19 : BusSelector  OutputSignals=VOUTP_SHA4_cnt
  bus_selector2 : BusSelector  OutputSignals=VOUTP_HWVer3_cnt
  bus_selector20 : BusSelector  OutputSignals=VOUTP_SHA5_cnt
  bus_selector21 : BusSelector  OutputSignals=VOUTP_SHA6_cnt
  bus_selector22 : BusSelector  OutputSignals=VOUTP_SHA7_cnt
  bus_selector23 : BusSelector  OutputSignals=VOUTP_SHA8_cnt
  bus_selector24 : BusSelector  OutputSignals=VOUTP_Variation_cnt
  bus_selector25 : BusSelector  OutputSignals=VOUTP_Change1_cnt
  bus_selector26 : BusSelector  OutputSignals=VOUTP_Change2_cnt
  bus_selector27 : BusSelector  OutputSignals=VOUTP_Dash1_cnt
  bus_selector28 : BusSelector  OutputSignals=VOUTP_Dash2_cnt
  bus_selector3 : BusSelector  OutputSignals=VOUTP_CarModel1_cnt
  bus_selector4 : BusSelector  OutputSignals=VOUTP_CarModel2_cnt
  bus_selector5 : BusSelector  OutputSignals=VOUTP_CarModel3_cnt
  bus_selector6 : BusSelector  OutputSignals=VOUTP_ECU1_cnt
  bus_selector7 : BusSelector  OutputSignals=VOUTP_ECU2_cnt
  bus_selector8 : BusSelector  OutputSignals=VOUTP_Country1_cnt
  bus_selector9 : BusSelector  OutputSignals=VOUTP_Country2_cnt
  FD2_Version : Outport
  wires:
  BSCP_outputs/1 -> [BSCP_outputs]
  BOUTP_outputs/1 -> [BOUTP_outputs]
  [CAN2_FUSION_HW_Ver1] -> bus_creator/1  "CAN2_FUSION_HW_Ver1"
  [CAN2_FUSION_HW_Ver2] -> bus_creator/2  "CAN2_FUSION_HW_Ver2"
  [CAN2_FUSION_HW_Ver3] -> bus_creator/3  "CAN2_FUSION_HW_Ver3"
  [CAN2_FUSION_SW_CarModel1] -> bus_creator/4  "CAN2_FUSION_SW_CarModel1"
  [CAN2_FUSION_SW_CarModel2] -> bus_creator/5  "CAN2_FUSION_SW_CarModel2"
  [CAN2_FUSION_SW_CarModel3] -> bus_creator/6  "CAN2_FUSION_SW_CarModel3"
  [CAN2_FUSION_SW_Controller1] -> bus_creator/7  "CAN2_FUSION_SW_Controller1"
  [CAN2_FUSION_SW_Controller2] -> bus_creator/8  "CAN2_FUSION_SW_Controller2"
  [CAN2_FUSION_SW_Country1] -> bus_creator/9  "CAN2_FUSION_SW_Country1"
  [CAN2_FUSION_SW_Country2] -> bus_creator/10  "CAN2_FUSION_SW_Country2"
  [CAN2_FUSION_SW_ECUGen1] -> bus_creator/11  "CAN2_FUSION_SW_ECUGen1"
  [CAN2_FUSION_SW_ECUGen2] -> bus_creator/12  "CAN2_FUSION_SW_ECUGen2"
  [CAN2_FUSION_SW_Major1] -> bus_creator/13  "CAN2_FUSION_SW_Major1"
  [CAN2_FUSION_SW_Major2] -> bus_creator/14  "CAN2_FUSION_SW_Major2"
  [CAN2_FUSION_SW_Minor1] -> bus_creator/15  "CAN2_FUSION_SW_Minor1"
  [CAN2_FUSION_SW_Minor2] -> bus_creator/16  "CAN2_FUSION_SW_Minor2"
  [CAN2_FUSION_SW_Patch1] -> bus_creator/17  "CAN2_FUSION_SW_Patch1"
  [CAN2_FUSION_SW_Patch2] -> bus_creator/18  "CAN2_FUSION_SW_Patch2"
  [CAN2_FUSION_SW_SHA1] -> bus_creator/19  "CAN2_FUSION_SW_SHA1"
  [CAN2_FUSION_SW_SHA2] -> bus_creator/20  "CAN2_FUSION_SW_SHA2"
  [CAN2_FUSION_SW_SHA3] -> bus_creator/21  "CAN2_FUSION_SW_SHA3"
  [CAN2_FUSION_SW_SHA4] -> bus_creator/22  "CAN2_FUSION_SW_SHA4"
  [CAN2_FUSION_SW_SHA5] -> bus_creator/23  "CAN2_FUSION_SW_SHA5"
  [CAN2_FUSION_SW_SHA6] -> bus_creator/24  "CAN2_FUSION_SW_SHA6"
  [CAN2_FUSION_SW_SHA7] -> bus_creator/25  "CAN2_FUSION_SW_SHA7"
  [CAN2_FUSION_SW_SHA8] -> bus_creator/26  "CAN2_FUSION_SW_SHA8"
  [CAN2_FUSION_SW_Var1] -> bus_creator/27  "CAN2_FUSION_SW_Var1"
  [CAN2_FUSION_SW_Var2] -> bus_creator/28  "CAN2_FUSION_SW_Var2"
  [CAN2_FUSION_SW_Var3] -> bus_creator/29  "CAN2_FUSION_SW_Var3"
  [CAN2_FUSION_SW_Var4] -> bus_creator/30  "CAN2_FUSION_SW_Var4"
  [CAN2_FUSION_SW_Var5] -> bus_creator/31  "CAN2_FUSION_SW_Var5"
  [CAN2_FUSION_SW_change1] -> bus_creator/32  "CAN2_FUSION_SW_change1"
  [CAN2_FUSION_SW_change2] -> bus_creator/33  "CAN2_FUSION_SW_change2"
  [CAN2_FUSION_SW_dash1] -> bus_creator/34  "CAN2_FUSION_SW_dash1"
  [CAN2_FUSION_SW_dash2] -> bus_creator/35  "CAN2_FUSION_SW_dash2"
  bus_creator/1 -> FD2_Version/1
  FUSIONHWVer1/1(CAN2_FUSION_HW_Ver1) -> [CAN2_FUSION_HW_Ver1]
  FUSIONHWVer2/1(CAN2_FUSION_HW_Ver2) -> [CAN2_FUSION_HW_Ver2]
  FUSIONHWVer3/1(CAN2_FUSION_HW_Ver3) -> [CAN2_FUSION_HW_Ver3]
  FUSIONSWCarModel1/1(CAN2_FUSION_SW_CarModel1) -> [CAN2_FUSION_SW_CarModel1]
  FUSIONSWCarModel2/1(CAN2_FUSION_SW_CarModel2) -> [CAN2_FUSION_SW_CarModel2]
  FUSIONSWCarModel3/1(CAN2_FUSION_SW_CarModel3) -> [CAN2_FUSION_SW_CarModel3]
  FUSIONSWController1/1(CAN2_FUSION_SW_Controller1) -> [CAN2_FUSION_SW_Controller1]
  FUSIONSWController2/1(CAN2_FUSION_SW_Controller2) -> [CAN2_FUSION_SW_Controller2]
  FUSIONSWCountry1/1(CAN2_FUSION_SW_Country1) -> [CAN2_FUSION_SW_Country1]
  FUSIONSWCountry2/1(CAN2_FUSION_SW_Country2) -> [CAN2_FUSION_SW_Country2]
  FUSIONSWECUGen1/1(CAN2_FUSION_SW_ECUGen1) -> [CAN2_FUSION_SW_ECUGen1]
  FUSIONSWECUGen2/1(CAN2_FUSION_SW_ECUGen2) -> [CAN2_FUSION_SW_ECUGen2]
  FUSIONSWMajor1/1(CAN2_FUSION_SW_Major1) -> [CAN2_FUSION_SW_Major1]
  FUSIONSWMajor2/1(CAN2_FUSION_SW_Major2) -> [CAN2_FUSION_SW_Major2]
  FUSIONSWMinor1/1(CAN2_FUSION_SW_Minor1) -> [CAN2_FUSION_SW_Minor1]
  FUSIONSWMinor2/1(CAN2_FUSION_SW_Minor2) -> [CAN2_FUSION_SW_Minor2]
  FUSIONSWPatch1/1(CAN2_FUSION_SW_Patch1) -> [CAN2_FUSION_SW_Patch1]
  FUSIONSWPatch2/1(CAN2_FUSION_SW_Patch2) -> [CAN2_FUSION_SW_Patch2]
  FUSIONSWSHA1/1(CAN2_FUSION_SW_SHA1) -> [CAN2_FUSION_SW_SHA1]
  FUSIONSWSHA2/1(CAN2_FUSION_SW_SHA2) -> [CAN2_FUSION_SW_SHA2]
  FUSIONSWSHA3/1(CAN2_FUSION_SW_SHA3) -> [CAN2_FUSION_SW_SHA3]
  FUSIONSWSHA4/1(CAN2_FUSION_SW_SHA4) -> [CAN2_FUSION_SW_SHA4]
  FUSIONSWSHA5/1(CAN2_FUSION_SW_SHA5) -> [CAN2_FUSION_SW_SHA5]
  FUSIONSWSHA6/1(CAN2_FUSION_SW_SHA6) -> [CAN2_FUSION_SW_SHA6]
  FUSIONSWSHA7/1(CAN2_FUSION_SW_SHA7) -> [CAN2_FUSION_SW_SHA7]
  FUSIONSWSHA8/1(CAN2_FUSION_SW_SHA8) -> [CAN2_FUSION_SW_SHA8]
  FUSIONSWVar1/1(CAN2_FUSION_SW_Var1) -> [CAN2_FUSION_SW_Var1]
  FUSIONSWVar2/1(CAN2_FUSION_SW_Var2) -> [CAN2_FUSION_SW_Var2]
  FUSIONSWVar3/1(CAN2_FUSION_SW_Var3) -> [CAN2_FUSION_SW_Var3]
  FUSIONSWVar4/1(CAN2_FUSION_SW_Var4) -> [CAN2_FUSION_SW_Var4]
  FUSIONSWVar5/1(CAN2_FUSION_SW_Var5) -> [CAN2_FUSION_SW_Var5]
  FUSIONSWchange1/1(CAN2_FUSION_SW_change1) -> [CAN2_FUSION_SW_change1]
  FUSIONSWchange2/1(CAN2_FUSION_SW_change2) -> [CAN2_FUSION_SW_change2]
  FUSIONSWdash1/1(CAN2_FUSION_SW_dash1) -> [CAN2_FUSION_SW_dash1]
  FUSIONSWdash2/1(CAN2_FUSION_SW_dash2) -> [CAN2_FUSION_SW_dash2]
  bus_selector/1 -> FUSIONHWVer1/1(FUSIONHWVer1)  "<VOUTP_HWVer1_cnt>"
  [BOUTP_outputs] -> bus_selector/1
  bus_selector1/1 -> FUSIONHWVer2/1(FUSIONHWVer2)  "<VOUTP_HWVer2_cnt>"
  [BOUTP_outputs] -> bus_selector1/1
  bus_selector2/1 -> FUSIONHWVer3/1(FUSIONHWVer3)  "<VOUTP_HWVer3_cnt>"
  [BOUTP_outputs] -> bus_selector2/1
  bus_selector3/1 -> FUSIONSWCarModel1/1(FUSIONSWCarModel1)  "<VOUTP_CarModel1_cnt>"
  [BOUTP_outputs] -> bus_selector3/1
  bus_selector4/1 -> FUSIONSWCarModel2/1(FUSIONSWCarModel2)  "<VOUTP_CarModel2_cnt>"
  [BOUTP_outputs] -> bus_selector4/1
  bus_selector5/1 -> FUSIONSWCarModel3/1(FUSIONSWCarModel3)  "<VOUTP_CarModel3_cnt>"
  [BOUTP_outputs] -> bus_selector5/1
  bus_selector6/1 -> FUSIONSWController1/1(FUSIONSWController1)  "<VOUTP_ECU1_cnt>"
  [BOUTP_outputs] -> bus_selector6/1
  bus_selector7/1 -> FUSIONSWController2/1(FUSIONSWController2)  "<VOUTP_ECU2_cnt>"
  [BOUTP_outputs] -> bus_selector7/1
  bus_selector8/1 -> FUSIONSWCountry1/1(FUSIONSWCountry1)  "<VOUTP_Country1_cnt>"
  [BOUTP_outputs] -> bus_selector8/1
  bus_selector9/1 -> FUSIONSWCountry2/1(FUSIONSWCountry2)  "<VOUTP_Country2_cnt>"
  [BOUTP_outputs] -> bus_selector9/1
  Ground/1 -> FUSIONSWECUGen1/1(FUSIONSWECUGen1)
  Ground1/1 -> FUSIONSWECUGen2/1(FUSIONSWECUGen2)
  bus_selector10/1 -> FUSIONSWMajor1/1(FUSIONSWMajor1)  "<VOUTP_Major1_cnt>"
  [BOUTP_outputs] -> bus_selector10/1
  bus_selector11/1 -> FUSIONSWMajor2/1(FUSIONSWMajor2)  "<VOUTP_Major2_cnt>"
  [BOUTP_outputs] -> bus_selector11/1
  bus_selector12/1 -> FUSIONSWMinor1/1(FUSIONSWMinor1)  "<VOUTP_Minor1_cnt>"
  [BOUTP_outputs] -> bus_selector12/1
  bus_selector13/1 -> FUSIONSWMinor2/1(FUSIONSWMinor2)  "<VOUTP_Minor2_cnt>"
  [BOUTP_outputs] -> bus_selector13/1
  bus_selector14/1 -> FUSIONSWPatch1/1(FUSIONSWPatch1)  "<VOUTP_Patch1_cnt>"
  [BOUTP_outputs] -> bus_selector14/1
  bus_selector15/1 -> FUSIONSWPatch2/1(FUSIONSWPatch2)  "<VOUTP_Patch2_cnt>"
  [BOUTP_outputs] -> bus_selector15/1
  bus_selector16/1 -> FUSIONSWSHA1/1(FUSIONSWSHA1)  "<VOUTP_SHA1_cnt>"
  [BOUTP_outputs] -> bus_selector16/1
  bus_selector17/1 -> FUSIONSWSHA2/1(FUSIONSWSHA2)  "<VOUTP_SHA2_cnt>"
  [BOUTP_outputs] -> bus_selector17/1
  bus_selector18/1 -> FUSIONSWSHA3/1(FUSIONSWSHA3)  "<VOUTP_SHA3_cnt>"
  [BOUTP_outputs] -> bus_selector18/1
  bus_selector19/1 -> FUSIONSWSHA4/1(FUSIONSWSHA4)  "<VOUTP_SHA4_cnt>"
  [BOUTP_outputs] -> bus_selector19/1
  bus_selector20/1 -> FUSIONSWSHA5/1(FUSIONSWSHA5)  "<VOUTP_SHA5_cnt>"
  [BOUTP_outputs] -> bus_selector20/1
  bus_selector21/1 -> FUSIONSWSHA6/1(FUSIONSWSHA6)  "<VOUTP_SHA6_cnt>"
  [BOUTP_outputs] -> bus_selector21/1
  bus_selector22/1 -> FUSIONSWSHA7/1(FUSIONSWSHA7)  "<VOUTP_SHA7_cnt>"
  [BOUTP_outputs] -> bus_selector22/1
  bus_selector23/1 -> FUSIONSWSHA8/1(FUSIONSWSHA8)  "<VOUTP_SHA8_cnt>"
  [BOUTP_outputs] -> bus_selector23/1
  bus_selector24/1 -> FUSIONSWVar1/1(FUSIONSWVar1)  "<VOUTP_Variation_cnt>"
  [BOUTP_outputs] -> bus_selector24/1
  Ground2/1 -> FUSIONSWVar2/1(FUSIONSWVar2)
  Ground3/1 -> FUSIONSWVar3/1(FUSIONSWVar3)
  Ground4/1 -> FUSIONSWVar4/1(FUSIONSWVar4)
  Ground5/1 -> FUSIONSWVar5/1(FUSIONSWVar5)
  bus_selector25/1 -> FUSIONSWchange1/1(FUSIONSWchange1)  "<VOUTP_Change1_cnt>"
  [BOUTP_outputs] -> bus_selector25/1
  bus_selector26/1 -> FUSIONSWchange2/1(FUSIONSWchange2)  "<VOUTP_Change2_cnt>"
  [BOUTP_outputs] -> bus_selector26/1
  bus_selector27/1 -> FUSIONSWdash1/1(FUSIONSWdash1)  "<VOUTP_Dash1_cnt>"
  [BOUTP_outputs] -> bus_selector27/1
  bus_selector28/1 -> FUSIONSWdash2/1(FUSIONSWdash2)  "<VOUTP_Dash2_cnt>"
  [BOUTP_outputs] -> bus_selector28/1

== system halout/HAL_OUT/CAN2/GW2_CE100_0_0x1C2 ==
  BSCP_outputs : Inport  OutDataTypeStr=Bus: BSCP_outputs
  BOUTP_outputs : Inport  Port=2  OutDataTypeStr=Bus: BOUTP_outputs
  FDCBCMDimSw : Subsystem
  FDCBCMFWipSwSta : Subsystem
  FDCBCMTurnSwSta : Subsystem
  bus_creator : BusCreator  Inputs=3  OutDataTypeStr=Bus: DT_CAN2_SG_GW2_CE100_0  NonVirtualBus=on
  bus_selector : BusSelector  OutputSignals=VOUTP_DimSwSta_flg
  bus_selector1 : BusSelector  OutputSignals=VOUTP_FWipSwSta_enum
  bus_selector2 : BusSelector  OutputSignals=VOUTP_TurnSwSta_enum
  GW2_CE100_0 : Outport
  wires:
  BSCP_outputs/1 -> [BSCP_outputs]
  BOUTP_outputs/1 -> [BOUTP_outputs]
  [CAN2_FDC_BCM_DimSw] -> bus_creator/1  "CAN2_FDC_BCM_DimSw"
  [CAN2_FDC_BCM_FWipSw_Sta] -> bus_creator/2  "CAN2_FDC_BCM_FWipSw_Sta"
  [CAN2_FDC_BCM_TurnSw_Sta] -> bus_creator/3  "CAN2_FDC_BCM_TurnSw_Sta"
  bus_creator/1 -> GW2_CE100_0/1
  FDCBCMDimSw/1(CAN2_FDC_BCM_DimSw) -> [CAN2_FDC_BCM_DimSw]
  FDCBCMFWipSwSta/1(CAN2_FDC_BCM_FWipSw_Sta) -> [CAN2_FDC_BCM_FWipSw_Sta]
  FDCBCMTurnSwSta/1(CAN2_FDC_BCM_TurnSw_Sta) -> [CAN2_FDC_BCM_TurnSw_Sta]
  bus_selector/1 -> FDCBCMDimSw/1(FDCBCMDimSw)  "<VOUTP_DimSwSta_flg>"
  [BOUTP_outputs] -> bus_selector/1
  bus_selector1/1 -> FDCBCMFWipSwSta/1(FDCBCMFWipSwSta)  "<VOUTP_FWipSwSta_enum>"
  [BOUTP_outputs] -> bus_selector1/1
  bus_selector2/1 -> FDCBCMTurnSwSta/1(FDCBCMTurnSwSta)  "<VOUTP_TurnSwSta_enum>"
  [BOUTP_outputs] -> bus_selector2/1
